simulink model "model_scc"  (R2013b)
settings: Solver=ode45  StartTime=0.0  StopTime=10.0  RelTol=1e-3
libraries: simulink x2
settings Model: Creator=IVDL  LastModifiedBy=edward
settings DataIOCC: SignalLoggingSaveFormat=ModelDataLogs
settings DebuggingCC: UnderspecifiedInitializationDetection=Simplified  MultiTaskDSMMsg=warning  MultiTaskCondExecSysMsg=none  StrictBusMsg=None
settings RTWCC: IncludeERTFirstTime=on
settings GRTTargetCC: CodeReplacementLibrary=None  CPPClassGenCompliant=on

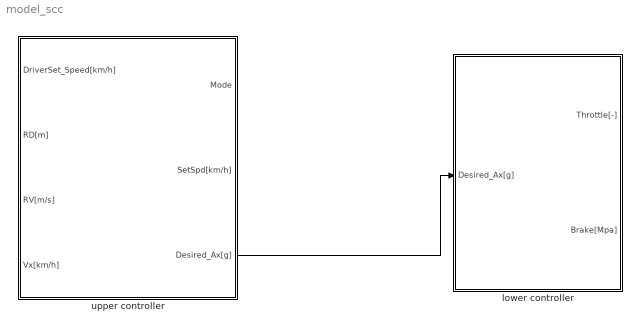
== system model_scc ==
  lower controller : Subsystem
  upper controller : Subsystem
  wires:
  upper controller/3(Desired_Ax[g]) -> lower controller/1(Desired_Ax[g])

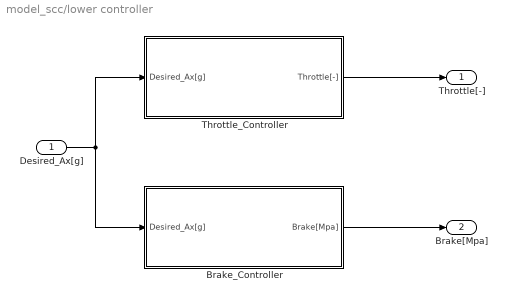
== system model_scc/lower controller ==
  Desired_Ax[g] : Inport
  Brake_Controller : Subsystem
  Throttle_Controller : Subsystem
  Throttle[-] : Outport
  Brake[Mpa] : Outport  Port=2
  wires:
  Desired_Ax[g]/1 -> Throttle_Controller/1(Desired_Ax[g]), Brake_Controller/1(Desired_Ax[g])
  Throttle_Controller/1(Throttle[-]) -> Throttle[-]/1
  Brake_Controller/1(Brake[Mpa]) -> Brake[Mpa]/1

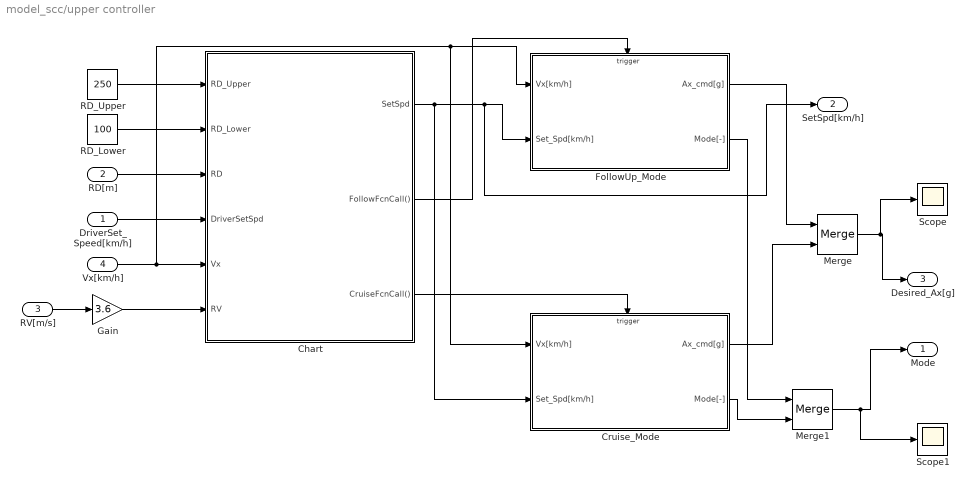
== system model_scc/upper controller ==
  DriverSet_Speed[km/h] : Inport
  RD[m] : Inport  Port=2
  RV[m/s] : Inport  Port=3
  Vx[km/h] : Inport  Port=4
  Chart : Stateflow chart  TreatAsAtomicUnit=on
  Cruise_Mode : Subsystem  TreatAsAtomicUnit=on
  FollowUp_Mode : Subsystem  TreatAsAtomicUnit=on
  Gain : Gain  Gain=3.6
  Merge : Merge
  Merge1 : Merge
  RD_Lower : Constant  Value=100
  RD_Upper : Constant  Value=250
  Scope : Scope
  Scope1 : Scope
  Mode : Outport
  SetSpd[km/h] : Outport  Port=2
  Desired_Ax[g] : Outport  Port=3
  wires:
  RD[m]/1 -> Chart/3(RD)
  RV[m/s]/1 -> Gain/1
  Vx[km/h]/1 -> Cruise_Mode/1(Vx[km/h]), FollowUp_Mode/1(Vx[km/h]), Chart/5(Vx)
  DriverSet_Speed[km/h]/1 -> Chart/4(DriverSetSpd)
  Gain/1 -> Chart/6(RV)
  RD_Upper/1 -> Chart/1(RD_Upper)
  RD_Lower/1 -> Chart/2(RD_Lower)
  Chart/3(CruiseFcnCall()) -> Cruise_Mode/Trigger
  Chart/2(FollowFcnCall()) -> FollowUp_Mode/Trigger
  Chart/1(SetSpd) -> Cruise_Mode/2(Set_Spd[km/h]), SetSpd[km/h]/1, FollowUp_Mode/2(Set_Spd[km/h])
  FollowUp_Mode/1(Ax_cmd[g]) -> Merge/1
  Cruise_Mode/1(Ax_cmd[g]) -> Merge/2
  Merge/1 -> Scope/1, Desired_Ax[g]/1
  FollowUp_Mode/2(Mode[-]) -> Merge1/1
  Cruise_Mode/2(Mode[-]) -> Merge1/2
  Merge1/1 -> Scope1/1, Mode/1

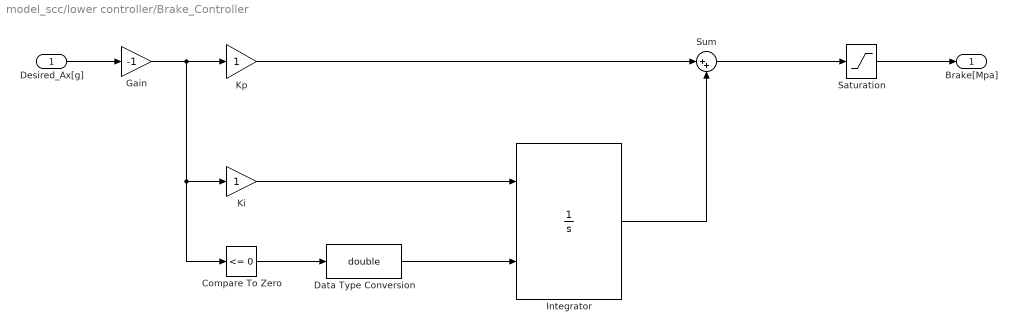
== system model_scc/lower controller/Brake_Controller ==
  Desired_Ax[g] : Inport
  Compare To Zero : simulink/Logic and Bit Operations/Compare To Zero  relop=<=  OutDataTypeStr=boolean
  Data Type Conversion : DataTypeConversion  OutDataTypeStr=double
  Gain : Gain  Gain=-1
  Integrator : Integrator  ExternalReset=rising
  Ki : Gain
  Kp : Gain
  Saturation : Saturate  UpperLimit=6  LowerLimit=0
  Sum : Sum  Inputs=|++
  Brake[Mpa] : Outport
  wires:
  Compare To Zero/1 -> Data Type Conversion/1
  Data Type Conversion/1 -> Integrator/2
  Ki/1 -> Integrator/1
  Integrator/1 -> Sum/2
  Kp/1 -> Sum/1
  Desired_Ax[g]/1 -> Gain/1
  Sum/1 -> Saturation/1
  Saturation/1 -> Brake[Mpa]/1
  Gain/1 -> Compare To Zero/1, Ki/1, Kp/1

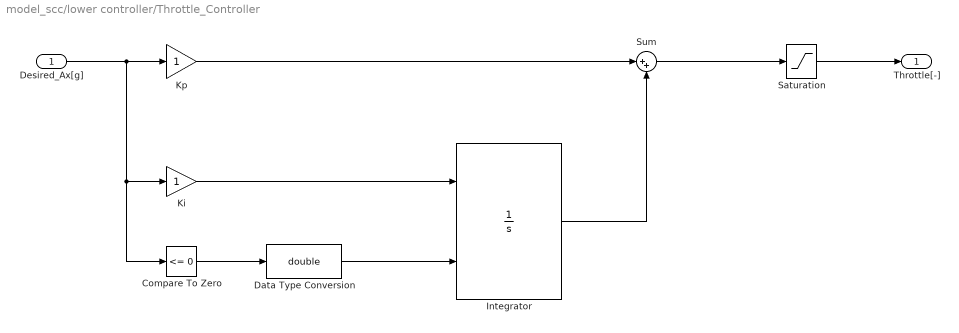
== system model_scc/lower controller/Throttle_Controller ==
  Desired_Ax[g] : Inport
  Compare To Zero : simulink/Logic and Bit Operations/Compare To Zero  relop=<=  OutDataTypeStr=boolean
  Data Type Conversion : DataTypeConversion  OutDataTypeStr=double
  Integrator : Integrator  ExternalReset=rising
  Ki : Gain
  Kp : Gain
  Saturation : Saturate  UpperLimit=1  LowerLimit=0
  Sum : Sum  Inputs=|++
  Throttle[-] : Outport
  wires:
  Compare To Zero/1 -> Data Type Conversion/1
  Data Type Conversion/1 -> Integrator/2
  Ki/1 -> Integrator/1
  Integrator/1 -> Sum/2
  Kp/1 -> Sum/1
  Desired_Ax[g]/1 -> Compare To Zero/1, Ki/1, Kp/1
  Sum/1 -> Saturation/1
  Saturation/1 -> Throttle[-]/1

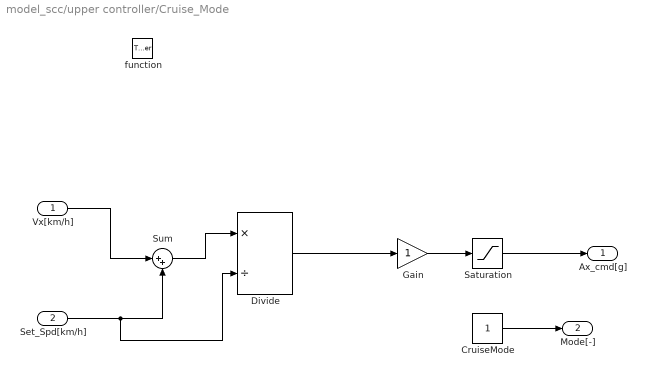
== system model_scc/upper controller/Cruise_Mode ==
  Vx[km/h] : Inport
  Set_Spd[km/h] : Inport  Port=2
  function : TriggerPort  TriggerType=function-call
  CruiseMode : Constant
  Divide : Product  Inputs=*/
  Gain : Gain
  Saturation : Saturate  UpperLimit=0.4  LowerLimit=-0.4
  Sum : Sum  Inputs=|++
  Ax_cmd[g] : Outport
  Mode[-] : Outport  Port=2
  wires:
  Set_Spd[km/h]/1 -> Divide/2, Sum/2
  Vx[km/h]/1 -> Sum/1
  Sum/1 -> Divide/1
  Divide/1 -> Gain/1
  Gain/1 -> Saturation/1
  CruiseMode/1 -> Mode[-]/1
  Saturation/1 -> Ax_cmd[g]/1

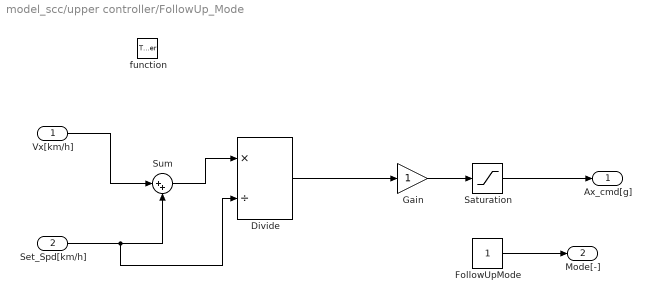
== system model_scc/upper controller/FollowUp_Mode ==
  Vx[km/h] : Inport
  Set_Spd[km/h] : Inport  Port=2
  function : TriggerPort  TriggerType=function-call
  Divide : Product  Inputs=*/
  FollowUpMode : Constant
  Gain : Gain
  Saturation : Saturate  UpperLimit=0.4  LowerLimit=-0.4
  Sum : Sum  Inputs=|++
  Ax_cmd[g] : Outport
  Mode[-] : Outport  Port=2
  wires:
  Set_Spd[km/h]/1 -> Divide/2, Sum/2
  Vx[km/h]/1 -> Sum/1
  Sum/1 -> Divide/1
  Divide/1 -> Gain/1
  Gain/1 -> Saturation/1
  FollowUpMode/1 -> Mode[-]/1
  Saturation/1 -> Ax_cmd[g]/1

== stateflow chart model_scc/upper controller/Chart ==
  state FollowUp_Mode
    du, en : TVSpd=RV+Vx;
    du : send(FollowFcnCall);
    du : SetSpd=TVSpd;
  state Cruise_Mode
    du, en : TVSpd=RV+Vx;
    du : send(CruiseFcnCall);
    du : SetSpd=DriverSetSpd;
  (default) -> Cruise_Mode
  Cruise_Mode -> FollowUp_Mode : [(RD<=RD_Lower) & (DriverSetSpd>=TVSpd)]
  FollowUp_Mode -> Cruise_Mode : [(RD>RD_Upper) | (DriverSetSpd<TVSpd)]
  data: RD_Upper input double; RD_Lower input double; RD input double; DriverSetSpd input double; Vx input double; RV input double; SetSpd output double; TVSpd local double
  events: FollowFcnCall output FUNCTION_CALL_EVENT; CruiseFcnCall output FUNCTION_CALL_EVENT
